simulink model "boost"  (Simulink 7.3)
settings: Solver=ode45  StartTime=0.0  StopTime=1  RelTol=1e-3
undefined symbols (not defined in the file): Hydride, Metal, Nickel
libraries: powerlib x15, simulink x6, powerlib_models x4, electricdrivelib x2, powerlib_extras x2
settings Model: Creator=lenovo  LastModifiedBy=Gireesh

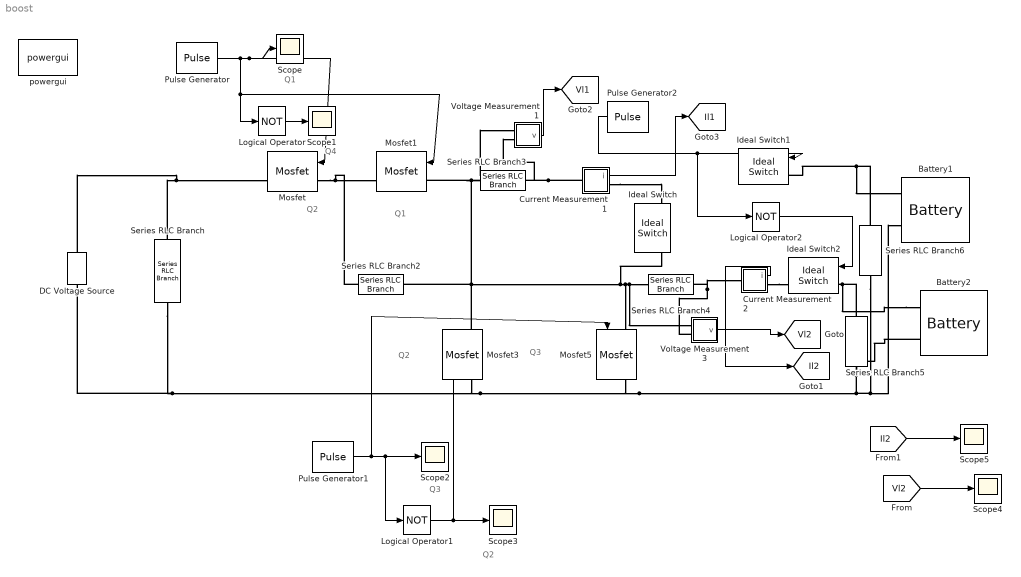
== system boost ==
  note: Q1
  note: Q4
  note: Q1
  note: Q2
  note: Q3
  note: Q2
  note: Q3
  note: Q2
  Battery1 : electricdrivelib/Extra Sources/Battery  SystemSampleTime=-1  BatType=Nickel-Metal-Hydride  ShowDetailedParameters=off  NomV=96  NomQ=1.5  SOC=100  PresetModel=on  MaxQ=1.6154  FullV=113.0847  Dis_rate=0.3  R=0.64  Normal_OP=1.4423  expZone="[104.1356           0.3]"  Dis_Char=off  current=[1.5 3]  Units=Ampere-hour  Batt_Tr=30
  Battery2 : electricdrivelib/Extra Sources/Battery  SystemSampleTime=-1  BatType=Nickel-Metal-Hydride  ShowDetailedParameters=off  NomV=48  NomQ=1.5  SOC=100  PresetModel=on  MaxQ=1.6154  FullV=56.5424  Dis_rate=0.3  R=0.32  Normal_OP=1.4423  expZone="[52.0678          0.3]"  Dis_Char=off  current=[1.5 3]  Units=Ampere-hour  Batt_Tr=30
  Current Measurement1 : Subsystem  DialogController=POWERSYS.PowerSysDialog  mask(Current Measurement){PhasorSimulation=off, OutputType=Complex, PSBequivalent=0}
      mask prompts: PhasorSimulation "Phasor simulation"; OutputType "Output signal :"; PSBequivalent "Equivalent circuit"
      mask help: Ideal current measurement.
      mask init:
      | block = gcb;
      | powericon('psbloadfunction',block,'Measurement Block','Initialize');
      | powericon('MeasurementBlockInit',block);
      | power_initmask();
      settings: CopyFcn=powericon('psbloadfunction',gcb,'Measurement Block','UpdateGotoTag');
      settings: PreSaveFcn=|
      | if strcmp('inactive',get_param(gcb,'linkstatus'));
      | 
      | set_param(gcb,'Linkstatus','restore')
      | end
      mask Help: web(psbhelp);
      mask StyleString: checkbox,popup(Complex|Real-Imag|Magnitude-Angle|Magnitude),edit
  Current Measurement2 : Subsystem  DialogController=POWERSYS.PowerSysDialog  mask(Current Measurement){PhasorSimulation=off, OutputType=Complex, PSBequivalent=0}
      mask prompts: PhasorSimulation "Phasor simulation"; OutputType "Output signal :"; PSBequivalent "Equivalent circuit"
      mask help: Ideal current measurement.
      mask init:
      | block = gcb;
      | powericon('psbloadfunction',block,'Measurement Block','Initialize');
      | powericon('MeasurementBlockInit',block);
      | power_initmask();
      settings: CopyFcn=powericon('psbloadfunction',gcb,'Measurement Block','UpdateGotoTag');
      settings: PreSaveFcn=|
      | if strcmp('inactive',get_param(gcb,'linkstatus'));
      | 
      | set_param(gcb,'Linkstatus','restore')
      | end
      mask Help: web(psbhelp);
      mask StyleString: checkbox,popup(Complex|Real-Imag|Magnitude-Angle|Magnitude),edit
  DC Voltage Source : powerlib/Electrical Sources/DC Voltage Source  DialogController=POWERSYS.PowerSysDialog  SystemSampleTime=-1  Amplitude=430  Measurements=None
  Ideal Switch : powerlib/Power Electronics/Ideal Switch  DialogController=POWERSYS.PowerSysDialog  SystemSampleTime=-1  Ron=0.001  Lon=0  IC=0  Rs=1e5  Cs=inf  Measurements=on
  Ideal Switch1 : powerlib/Power Electronics/Ideal Switch  DialogController=POWERSYS.PowerSysDialog  SystemSampleTime=-1  Ron=0.001  Lon=0  IC=0  Rs=1e5  Cs=inf  Measurements=on
  Ideal Switch2 : powerlib/Power Electronics/Ideal Switch  DialogController=POWERSYS.PowerSysDialog  SystemSampleTime=-1  Ron=0.001  Lon=0  IC=0  Rs=1e5  Cs=inf  Measurements=on
  Logical Operator : Logic  Operator=NOT  AllPortsSameDT=off  OutDataTypeMode=boolean  LogicDataType=fixdt(0, 8)  OutDataTypeStr=boolean
  Logical Operator1 : Logic  Operator=NOT  AllPortsSameDT=off  OutDataTypeMode=boolean  LogicDataType=fixdt(0, 8)  OutDataTypeStr=boolean
  Logical Operator2 : Logic  Operator=NOT  AllPortsSameDT=off  OutDataTypeMode=boolean  LogicDataType=fixdt(0, 8)  OutDataTypeStr=boolean
  Mosfet{,1,3,5} (4 alike) : powerlib/Power Electronics/Mosfet  DialogController=POWERSYS.PowerSysDialog  SystemSampleTime=-1  Ron=0.1  Lon=0  Rd=0.01  Vfd=0  IC=0  Rs=1e5  Cs=inf  Measurements=on
  Pulse Generator : DiscretePulseGenerator  PulseType=Time based  Amplitude=1  Period=0.02  PulseWidth=20  PhaseDelay=0  SampleTime=1
  Pulse Generator1 : DiscretePulseGenerator  PulseType=Time based  Amplitude=1  Period=0.02  PulseWidth=30  PhaseDelay=0  SampleTime=1
  Pulse Generator2 : DiscretePulseGenerator  PulseType=Time based  Amplitude=1  Period=0.02  PulseWidth=60  PhaseDelay=0  SampleTime=1
  Scope{,1..5} (6 alike) : Scope
      Scope2 settings: SaveName=ScopeData2
      Scope3 settings: SaveName=ScopeData3
      Scope4 settings: SaveName=ScopeData5
      Scope5 settings: SaveName=ScopeData6
  Series RLC Branch : powerlib/Elements/Series RLC Branch  DialogController=POWERSYS.PowerSysDialog  PhysicalDomain=powersysdomain  SubClassName=unknown  LeftPortType=p1  RightPortType=p1  LConnTagsString=__new0  RConnTagsString=__new0  BranchType=RC  Resistance=0.0001  Inductance=1e-3  SetiL0=off  InitialCurrent=0  Capacitance=1880e-6  Setx0=off  InitialVoltage=0  Measurements=None
  Series RLC Branch2 : powerlib/Elements/Series RLC Branch  DialogController=POWERSYS.PowerSysDialog  PhysicalDomain=powersysdomain  SubClassName=unknown  LeftPortType=p1  RightPortType=p1  LConnTagsString=__new0  RConnTagsString=__new0  BranchType=C  Resistance=1  Inductance=1e-3  SetiL0=off  InitialCurrent=0  Capacitance=400e-6  Setx0=off  InitialVoltage=0  Measurements=None
  Series RLC Branch3 : powerlib/Elements/Series RLC Branch  DialogController=POWERSYS.PowerSysDialog  PhysicalDomain=powersysdomain  SubClassName=unknown  LeftPortType=p1  RightPortType=p1  LConnTagsString=__new0  RConnTagsString=__new0  BranchType=L  Resistance=1  Inductance=250e-3  SetiL0=off  InitialCurrent=0  Capacitance=1e-6  Setx0=off  InitialVoltage=0  Measurements=None
  Series RLC Branch4 : powerlib/Elements/Series RLC Branch  DialogController=POWERSYS.PowerSysDialog  PhysicalDomain=powersysdomain  SubClassName=unknown  LeftPortType=p1  RightPortType=p1  LConnTagsString=__new0  RConnTagsString=__new0  BranchType=L  Resistance=1  Inductance=250e-3  SetiL0=off  InitialCurrent=0  Capacitance=1e-6  Setx0=off  InitialVoltage=0  Measurements=None
  Series RLC Branch5 : powerlib/Elements/Series RLC Branch  DialogController=POWERSYS.PowerSysDialog  PhysicalDomain=powersysdomain  SubClassName=unknown  LeftPortType=p1  RightPortType=p1  LConnTagsString=__new0  RConnTagsString=__new0  BranchType=C  Resistance=1  Inductance=1e-3  SetiL0=off  InitialCurrent=0  Capacitance=400e-6  Setx0=off  InitialVoltage=0  Measurements=None
  Series RLC Branch6 : powerlib/Elements/Series RLC Branch  DialogController=POWERSYS.PowerSysDialog  PhysicalDomain=powersysdomain  SubClassName=unknown  LeftPortType=p1  RightPortType=p1  LConnTagsString=__new0  RConnTagsString=__new0  BranchType=C  Resistance=1  Inductance=1e-3  SetiL0=off  InitialCurrent=0  Capacitance=400e-6  Setx0=off  InitialVoltage=0  Measurements=None
  Voltage Measurement1 : Subsystem  DialogController=POWERSYS.PowerSysDialog  mask(Voltage Measurement){PhasorSimulation=off, OutputType=Complex, PSBequivalent=0}
      mask prompts: PhasorSimulation "Phasor simulation"; OutputType "Output signal :"; PSBequivalent "Equivalent circuit"
      mask help: Ideal voltage measurement.
      mask init:
      | block = gcb;
      | powericon('psbloadfunction',block,'Measurement Block','Initialize');
      | powericon('MeasurementBlockInit',block);
      | power_initmask();
      settings: CopyFcn=powericon('psbloadfunction',gcb,'Measurement Block','UpdateGotoTag');
      settings: PreSaveFcn=|
      | if strcmp('inactive',get_param(gcb,'linkstatus'));
      | 
      | set_param(gcb,'Linkstatus','restore')
      | end
      mask Help: web(psbhelp);
      mask StyleString: checkbox,popup(Complex|Real-Imag|Magnitude-Angle|Magnitude),edit
  Voltage Measurement3 : Subsystem  DialogController=POWERSYS.PowerSysDialog  mask(Voltage Measurement){PhasorSimulation=off, OutputType=Complex, PSBequivalent=0}
      mask prompts: PhasorSimulation "Phasor simulation"; OutputType "Output signal :"; PSBequivalent "Equivalent circuit"
      mask help: Ideal voltage measurement.
      mask init:
      | block = gcb;
      | powericon('psbloadfunction',block,'Measurement Block','Initialize');
      | powericon('MeasurementBlockInit',block);
      | power_initmask();
      settings: CopyFcn=powericon('psbloadfunction',gcb,'Measurement Block','UpdateGotoTag');
      settings: PreSaveFcn=|
      | if strcmp('inactive',get_param(gcb,'linkstatus'));
      | 
      | set_param(gcb,'Linkstatus','restore')
      | end
      mask Help: web(psbhelp);
      mask StyleString: checkbox,popup(Complex|Real-Imag|Magnitude-Angle|Magnitude),edit
  powergui : powerlib/powergui  Priority=1  SystemSampleTime=-1  SimulationMode=Discrete  SampleTime=50e-6  frequency=60  SPID=off  DisableSnubberDevices=off  DisableRonSwitches=off  DisableVfSwitches=off  SwTol=0  Interpol=off  frequencyindice=0  echomessages=off  HookPort=off  DisplayEquations=off  FunctionMessages=off  EnableUseOfTLC=off  x0status=blocks  RestoreLinks=warning  Frange=[0:2:500]  Ylog=off  Xlog=on  ShowGrid=off  save=off  variable=ZData  ZoomFFT=on  StartTime=0.0  cycles=1  DisplayStyle=1  fundamental=60  FreqAxis=off  MaxFrequency=1000  frequencyindicesteady=1  RmsSteady=1  display=off  Ts=0  methode=off
  tag scope: Il1=global, Il2=global, Vl1=global, Vl2=global
  wires:
  Pulse Generator/1 -> Scope/1, Mosfet/1, Logical Operator/1, Mosfet1/1
  Logical Operator/1 -> Scope1/1
  Pulse Generator1/1 -> Scope2/1, Logical Operator1/1, Mosfet5/1
  Logical Operator1/1 -> Scope3/1, Mosfet3/1
  Pulse Generator2/1 -> Ideal Switch1/1, Logical Operator2/1
  Logical Operator2/1 -> Ideal Switch2/1
  Voltage Measurement3/1(v) -> [Vl2]
  [Vl2] -> Scope4/1
  [Il2] -> Scope5/1
  Current Measurement2/1(i) -> [Il2]
  Voltage Measurement1/1(v) -> [Vl1]
  Current Measurement1/1(i) -> [Il1]
  connections:
  Mosfet/LConn1 -- Mosfet1/RConn1 -- Series RLC Branch2/RConn1
  Series RLC Branch/LConn1 -- Mosfet/RConn1 -- DC Voltage Source/RConn1
  Series RLC Branch3/RConn1 -- Series RLC Branch4/RConn1 -- Voltage Measurement3/LConn1 -- Ideal Switch/RConn1 -- Mosfet5/LConn1 -- Mosfet3/LConn1 -- Series RLC Branch2/LConn1 -- Mosfet1/LConn1 -- Voltage Measurement1/LConn1
  Voltage Measurement3/LConn2 -- Series RLC Branch4/LConn1 -- Current Measurement2/LConn1
  Battery2/LConn1 -- Series RLC Branch5/LConn1 -- Ideal Switch2/LConn1
  Battery2/LConn2 -- Series RLC Branch5/RConn1 -- Series RLC Branch6/RConn1 -- Battery1/LConn2 -- Mosfet5/RConn1 -- Mosfet3/RConn1 -- Series RLC Branch/RConn1 -- DC Voltage Source/LConn1
  Ideal Switch1/LConn1 -- Battery1/LConn1 -- Series RLC Branch6/LConn1
  Current Measurement2/RConn1 -- Ideal Switch2/RConn1
  Current Measurement1/LConn1 -- Series RLC Branch3/LConn1 -- Voltage Measurement1/LConn2
  Current Measurement1/RConn1 -- Ideal Switch/LConn1

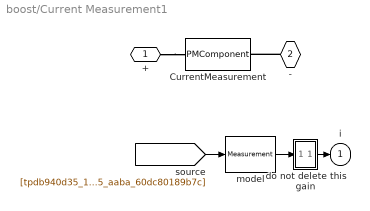
== system boost/Current Measurement1 ==
  CurrentMeasurement : PMComponent  PhysicalDomain=powersysdomain  LeftPortType=p1  RightPortType=p1  LConnTagsString=a  RConnTagsString=__new0
      mask Type: InnerPowersysBlock
  do not delete this gain : Subsystem  mask(Gain){x=1, XX=Element-wise(K.*u), Ts=50e-6}
      mask prompts: x "Gain"; XX "Muliplication"; Ts "Sample time(-1 for inherited)"
      mask help: Element-wise gain(y=K.*u)ot matrix gain(y=K*u or y=u*K).
      mask StyleString: edit,popup(Element-wise(K.*u)|Matrix(K*u)|Matrix(u*K)|Matrix(K*u(u vector)),edit
      mask Display:
      | plot([0 0 10 0],[0 10 5 0]);
      | disp('1  ')
  model : powerlib_models/Continuous/Measurement  SystemSampleTime=-1
  + : PMIOPort  Port=1  Side=Left
  - : PMIOPort  Port=2  Side=Right
  i : Outport  OutDataType=sfix(16)  OutScaling=2^0  InitialOutput=0
  wires:
  [tpdb940d35_1964_4865_aaba_60dc80189b7c] -> model/1
  model/1 -> do not delete this gain/1(In1)
  do not delete this gain/1(Out1) -> i/1
  connections:
  -/RConn1 -- CurrentMeasurement/RConn1
  +/RConn1 -- CurrentMeasurement/LConn1

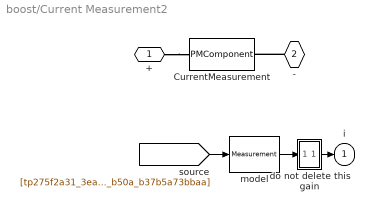
== system boost/Current Measurement2 ==
  CurrentMeasurement : PMComponent  PhysicalDomain=powersysdomain  LeftPortType=p1  RightPortType=p1  LConnTagsString=a  RConnTagsString=__new0
      mask Type: InnerPowersysBlock
  do not delete this gain : Subsystem  mask(Gain){x=1, XX=Element-wise(K.*u), Ts=50e-6}
      mask prompts: x "Gain"; XX "Muliplication"; Ts "Sample time(-1 for inherited)"
      mask help: Element-wise gain(y=K.*u)ot matrix gain(y=K*u or y=u*K).
      mask StyleString: edit,popup(Element-wise(K.*u)|Matrix(K*u)|Matrix(u*K)|Matrix(K*u(u vector)),edit
      mask Display:
      | plot([0 0 10 0],[0 10 5 0]);
      | disp('1  ')
  model : powerlib_models/Continuous/Measurement  SystemSampleTime=-1
  + : PMIOPort  Port=1  Side=Left
  - : PMIOPort  Port=2  Side=Right
  i : Outport  OutDataType=sfix(16)  OutScaling=2^0  InitialOutput=0
  wires:
  do not delete this gain/1(Out1) -> i/1
  model/1 -> do not delete this gain/1(In1)
  [tp275f2a31_3ea2_4c95_b50a_b37b5a73bbaa] -> model/1
  connections:
  +/RConn1 -- CurrentMeasurement/LConn1
  -/RConn1 -- CurrentMeasurement/RConn1

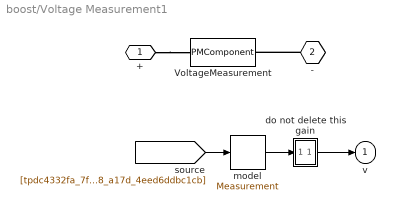
== system boost/Voltage Measurement1 ==
  VoltageMeasurement : PMComponent  PhysicalDomain=powersysdomain  LeftPortType=p1  RightPortType=p1  LConnTagsString=+  RConnTagsString=-
      mask Type: InnerPowersysBlock
  do not delete this gain : Subsystem  mask(Gain){x=1, XX=Element-wise(K.*u), Ts=0}
      mask prompts: x "Gain"; XX "Muliplication"; Ts "Sample time(-1 for inherited)"
      mask help: Eemnt-wise gain(y=K.*u)ot matrix gain(y=K*u or y=u*K).
      mask StyleString: edit,popup(Element-wise(K.*u)|Matrix(K*u)|Matrix(u*K)|Matrix(K*u(u vector)),edit
      mask Display:
      | plot([0 0 10 0],[0 10 5 0]);
      | disp('1')
  model : powerlib_models/Continuous/Measurement  SystemSampleTime=-1
  + : PMIOPort  Port=1  Side=Left
  - : PMIOPort  Port=2  Side=Left
  v : Outport  OutDataType=sfix(16)  OutScaling=2^0  InitialOutput=0
  wires:
  do not delete this gain/1(Out2) -> v/1
  model/1 -> do not delete this gain/1(In1)
  [tpdc4332fa_7f97_4f58_a17d_4eed6ddbc1cb] -> model/1
  connections:
  -/RConn1 -- VoltageMeasurement/RConn1
  +/RConn1 -- VoltageMeasurement/LConn1

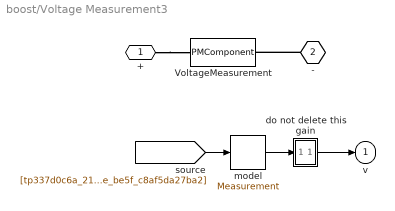
== system boost/Voltage Measurement3 ==
  VoltageMeasurement : PMComponent  PhysicalDomain=powersysdomain  LeftPortType=p1  RightPortType=p1  LConnTagsString=+  RConnTagsString=-
      mask Type: InnerPowersysBlock
  do not delete this gain : Subsystem  mask(Gain){x=1, XX=Element-wise(K.*u), Ts=0}
      mask prompts: x "Gain"; XX "Muliplication"; Ts "Sample time(-1 for inherited)"
      mask help: Eemnt-wise gain(y=K.*u)ot matrix gain(y=K*u or y=u*K).
      mask StyleString: edit,popup(Element-wise(K.*u)|Matrix(K*u)|Matrix(u*K)|Matrix(K*u(u vector)),edit
      mask Display:
      | plot([0 0 10 0],[0 10 5 0]);
      | disp('1')
  model : powerlib_models/Continuous/Measurement  SystemSampleTime=-1
  + : PMIOPort  Port=1  Side=Left
  - : PMIOPort  Port=2  Side=Left
  v : Outport  OutDataType=sfix(16)  OutScaling=2^0  InitialOutput=0
  wires:
  [tp337d0c6a_2107_40de_be5f_c8af5da27ba2] -> model/1
  model/1 -> do not delete this gain/1(In1)
  do not delete this gain/1(Out2) -> v/1
  connections:
  +/RConn1 -- VoltageMeasurement/LConn1
  -/RConn1 -- VoltageMeasurement/RConn1

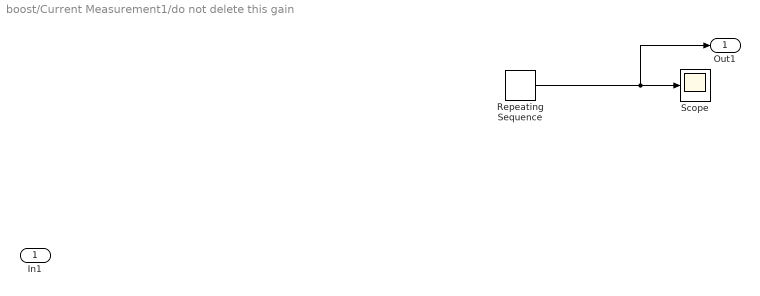
== system boost/Current Measurement1/do not delete this gain ==
  In1 : Inport  OutDataType=sfix(16)  OutScaling=2^0
  Repeating Sequence : simulink/Sources/Repeating Sequence  SystemSampleTime=-1  rep_seq_t=[0 0.02 0.04]  rep_seq_y=[0 6 0]
  Scope : Scope
      settings: TimeRange=1  SaveName=ScopeData7
  Out1 : Outport  OutDataType=sfix(16)  OutScaling=2^0
  wires:
  Repeating Sequence/1 -> Out1/1, Scope/1

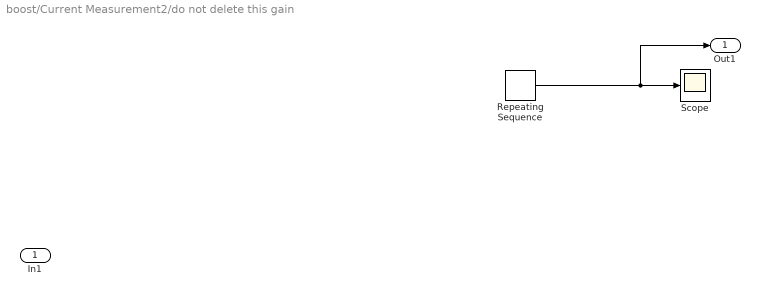
== system boost/Current Measurement2/do not delete this gain ==
  In1 : Inport  OutDataType=sfix(16)  OutScaling=2^0
  Repeating Sequence : simulink/Sources/Repeating Sequence  SystemSampleTime=-1  rep_seq_t=[0 0.02 0.04]  rep_seq_y=[0 6 0]
  Scope : Scope
      settings: TimeRange=1  SaveName=ScopeData7
  Out1 : Outport  OutDataType=sfix(16)  OutScaling=2^0
  wires:
  Repeating Sequence/1 -> Scope/1, Out1/1

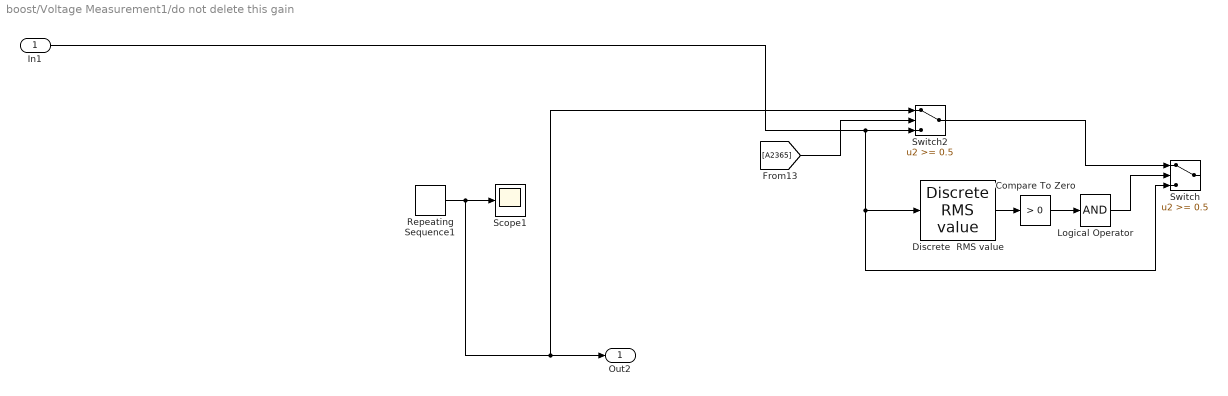
== system boost/Voltage Measurement1/do not delete this gain ==
  In1 : Inport  OutDataType=sfix(16)  OutScaling=2^0
  Compare To Zero : simulink/Logic and Bit Operations/Compare To Zero  SystemSampleTime=-1  relop=>  LogicOutDataTypeMode=uint8  ZeroCross=off
  Discrete  RMS value : powerlib_extras/Discrete Measurements/Discrete  RMS value  DialogController=POWERSYS.PowerSysDialog  SystemSampleTime=-1  Freq=60  Mag_Init=1  Ts=50e-6
  Logical Operator : Logic  Inputs=1  AllPortsSameDT=off  OutDataTypeMode=boolean  LogicDataType=fixdt(0, 8)  OutDataTypeStr=boolean
  Repeating Sequence1 : simulink/Sources/Repeating Sequence  SystemSampleTime=-1  rep_seq_t=[0 0.001 0.0011 0.0022 ]  rep_seq_y=[6 6 -6 -6]
  Scope1 : Scope
      settings: TimeRange=1  SaveName=ScopeData4
  Switch : Switch  Threshold=0.5  OutDataType=fixdt(1, 16)  OutScaling=2^0
  Switch2 : Switch  Threshold=0.5  OutDataType=fixdt(1, 16)  OutScaling=2^0
  Out2 : Outport  OutDataType=sfix(16)  OutScaling=2^0
  wires:
  Repeating Sequence1/1 -> Switch2/1, Out2/1, Scope1/1
  In1/1 -> Switch2/3, Discrete  RMS value/1, Switch/3
  ? -> ?
  [A2365] -> Switch2/2
  Switch2/1 -> Switch/1
  Discrete  RMS value/1 -> Compare To Zero/1
  Compare To Zero/1 -> Logical Operator/1
  Logical Operator/1 -> Switch/2

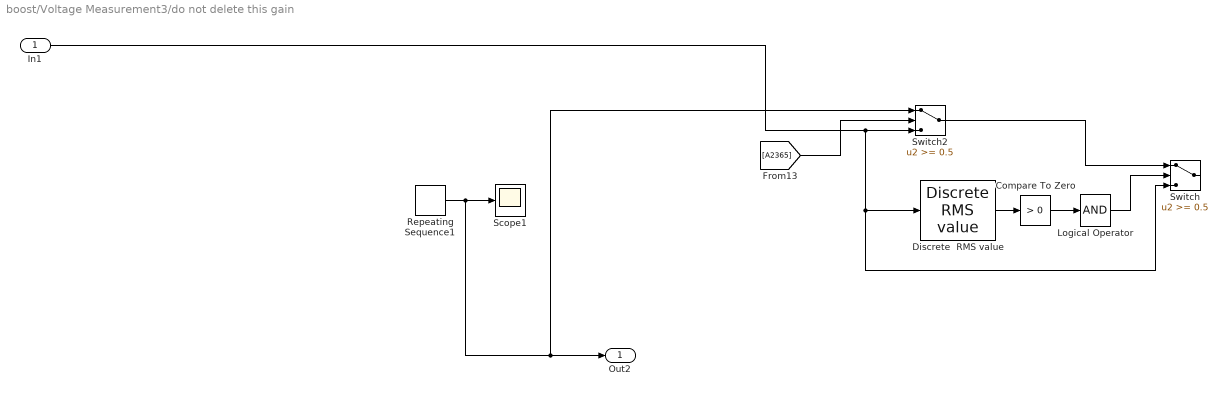
== system boost/Voltage Measurement3/do not delete this gain ==
  In1 : Inport  OutDataType=sfix(16)  OutScaling=2^0
  Compare To Zero : simulink/Logic and Bit Operations/Compare To Zero  SystemSampleTime=-1  relop=>  LogicOutDataTypeMode=uint8  ZeroCross=off
  Discrete  RMS value : powerlib_extras/Discrete Measurements/Discrete  RMS value  DialogController=POWERSYS.PowerSysDialog  SystemSampleTime=-1  Freq=60  Mag_Init=1  Ts=50e-6
  Logical Operator : Logic  Inputs=1  AllPortsSameDT=off  OutDataTypeMode=boolean  LogicDataType=fixdt(0, 8)  OutDataTypeStr=boolean
  Repeating Sequence1 : simulink/Sources/Repeating Sequence  SystemSampleTime=-1  rep_seq_t=[0 0.001 0.0011 0.0022 ]  rep_seq_y=[6 6 -6 -6]
  Scope1 : Scope
      settings: TimeRange=1  SaveName=ScopeData4
  Switch : Switch  Threshold=0.5  OutDataType=fixdt(1, 16)  OutScaling=2^0
  Switch2 : Switch  Threshold=0.5  OutDataType=fixdt(1, 16)  OutScaling=2^0
  Out2 : Outport  OutDataType=sfix(16)  OutScaling=2^0
  wires:
  Logical Operator/1 -> Switch/2
  Compare To Zero/1 -> Logical Operator/1
  Discrete  RMS value/1 -> Compare To Zero/1
  Switch2/1 -> Switch/1
  [A2365] -> Switch2/2
  ? -> ?
  In1/1 -> Switch/3, Discrete  RMS value/1, Switch2/3
  Repeating Sequence1/1 -> Scope1/1, Out2/1, Switch2/1
